simulink model "Control_test"  (R2014b)
settings: Solver=FixedStepDiscrete  StartTime=0.0  StopTime=Inf  FixedStep=0.001  RelTol=1e-3
PostLoadFcn:
  | , if any(exist('dsrtsu_mdlpostloadfcn', 'file') == [2, 3, 6]), try dsrtsu_mdlpostloadfcn('Execute', bdroot); catch fprintf('Error in PostLoadFcn (dsrtsu_mdlpostloadfcn) for model "%s":\n %s\n', bdroot, lasterr); end, end,
undefined symbols (not defined in the file or in its folder): dtLocal, slcm
libraries: rtican x163, simulink x14
(part 22 of 34)

== system Control_test/InputProcessing/RadarCanProcessing/Track24 ==
  Bus Creator : BusCreator  Inputs=12
  ESR_Track24 : rtican/RTICAN Receive (RX)   Reserved1=[]  Reserved2=[]  Reserved3=[]  Reserved4=[]  SfcnMessage=[]  Msg_Struct=[]  BoardTypeNo=[]  BoardNo=[]  ChannelNo=[]  Parameters=[]  DialogFcn=[]  UnitName=[]  Revision=[]  UnitValues=[]  DSProperties=struct('RTI',struct('Version',uint32(5),'BlockType',struct('isSLSource',uint8(1),'isSLSink',uint8(1),'isHWSource',uint8(0),'isHWSink',uint8(0),'isSetup',uint8(0),'isInline',uint8(1),'isNonInline',uint8(0),'isInterrupt',uint8(0),'isChannelwise',uint8(0)),'IOBoardType','RTICAN','UnitType','MESSAGE','Identifier','RX','DialogType','MSVC','BlockSet','RTICAN','SlaveProcessor','CAN'))  RTIBlockInterface=struct('OutputPortsWidth',int32([1 1 1 1 1 1 1 1 1 1 1 1]),'OutputPortsActive',[1 1 1 1 1 1 1 1 1 1 1 1],'OutputPortsName',{{'CAN_TX_TRACK_RANGE_RATE_24','CAN_TX_TRACK_MED_RANGE_MODE_24','CAN_TX_TRACK_RANGE_ACCEL_24','CAN_TX_TRACK_WIDTH_24','CAN_TX_TRACK_ROLLING_COUNT_24','CAN_TX_TRACK_BRIDGE_OBJECT_24','CAN_TX_TRACK_RANGE_24','CAN_TX_TRACK_ANGLE_24','CAN_TX_TRACK_STATUS_24','CAN_TX_TRACK_ONCOMING_24','CAN_TX_TRACK_GROUPING_CHANGED_24','CAN_TX_TRACK_LAT_RATE_24'}},'OutputPortsDataType',{{'SS_DOUBLE','SS_DOUBLE','SS_DOUBLE','SS_DOUBLE','SS_DOUBLE','SS_DOUBLE','SS_DOUBLE','SS_DOUBLE','SS_DOUBLE','SS_DOUBLE','SS_DOUBLE','SS_DOUBLE'}},'OutputPortsLabel',{{'CAN_TX_TRACK_RANGE_RATE_24','CAN_TX_TRACK_MED_RANGE_MODE_24','CAN_TX_TRACK_RANGE_ACCEL_24','CAN_TX_TRACK_WIDTH_24','CAN_TX_TRACK_ROLLING_COUNT_24','CAN_TX_TRACK_BRIDGE_OBJECT_24','CAN_TX_TRACK_RANGE_24','CAN_TX_TRACK_ANGLE_24','CAN_TX_TRACK_STATUS_24','CAN_TX_TRACK_ONCOMING_24','CAN_TX_TRACK_GROUPING_CHANGED_24','CAN_TX_TRACK_LAT_RATE_24'}},'OutputPortsLabelMode','ON','InputPortsWidth',int32(0),'InputPortsActive',0,'DialogFcn','rtican_message_interface_gui','BlockDisplay',{{'','center'}},'IconTransparency','on','ParameterTunableNames',{{}},'InitLevel',3,'BlockName',struct('Token',{{'ESR_Track24'}}),'SampleTime',{{0.01}},'TriggerPort',{{'none'}},'EnablePort',{{'none'}})  RTIBlockParameters=struct('BoardTypeNo',{{1,'OFF',[]}},'BoardNo',{{2,'ON',[1 16]}},'ChannelNo',{{2,'ON',[1 2]}},'Parameters',{{struct('DataFileSupport',struct('DataFileSelectedMaster',1,'DataFileSelectedLocal',0,'DataFileName','c:\users\mpc_car\documents\github\mpc-car\controller\dbcfiles\esr_dv3_64tgt.dbc|','DataFileDate',{{{['02-Nov-2012 20:32:52']},{['21-Mar-2013 13:39:53']},{['28-Sep-2011 17:08:52']}}},'SelectedFile',['<no file selected>'],'InterfaceFcn','rtican_dbc_file_parser'),'Options',struct('StatusSelected',0,'TimeSelected',0,'DeltaTimeSelected',0,'BytePortSelected',0,'MessageLengthSelected',0,'TriggerPort',struct('Selected',0,'TriggerType',0),'UserCoding',struct('Selected',0,'InterfaceFile','UserDecodingFile','FcnName','UserDecodeFcn','InportSelected',0,'InportWidth',1,'OutportSelected',0,'OutportWidth',1),'EnablePortSelected',0,'SignalOnPortnameSelected',1,'UseRXService',0),'Message',struct('MsgOnBlocknameSelected',1,'MsgName','ESR_Track24','MsgIdFormat',0,'MsgId',1303,'MsgLength',8,'NumSignals',12,'SampleTime',0.01,'Signal',struct('SgnName',{'CAN_TX_TRACK_RANGE_RATE_24','CAN_TX_TRACK_MED_RANGE_MODE_24','CAN_TX_TRACK_RANGE_ACCEL_24','CAN_TX_TRACK_WIDTH_24','CAN_TX_TRACK_ROLLING_COUNT_24','CAN_TX_TRACK_BRIDGE_OBJECT_24','CAN_TX_TRACK_RANGE_24','CAN_TX_TRACK_ANGLE_24','CAN_TX_TRACK_STATUS_24','CAN_TX_TRACK_ONCOMING_24','CAN_TX_TRACK_GROUPING_CHANGED_24','CAN_TX_TRACK_LAT_RATE_24'},'SgnStartBit',{0,14,16,26,30,31,32,43,53,56,57,58},'SgnLength',{14,2,10,4,1,1,11,10,3,1,1,6},'SgnType',{0,0,0,0,0,0,0,0,0,0,0,0},'ModeValue',{-1,-1,-1,-1,-1,-1,-1,-1,-1,-1,-1,-1},'DataType',{1,0,1,0,0,0,0,1,0,0,0,1},'ByteLayout',{2,2,2,2,2,2,2,2,2,2,2,2},'Factor',{0.01,1,0.05,0.5,1,1,0.1,0.1,1,1,1,0.25},'Offset',{0,0,0,0,0,0,0,0,0,0,0,0},'SgnComment',{{''},{''},{''},{''},{''},{''},{''},{''},{''},{''},{''},{''}},'SgnUnit',{'m/s','','m/s/s','m','','','m','deg','','','',''},'Min',{-81.92,0,-25.6,0,0,0,0,-51.2,0,0,0,-8},'Max',{81.91,3,25.55,7.5,1,0,204.7,51.1,7,0,0,7.75},'SLDataType',{'SS_DOUBLE','SS_DOUBLE','SS_DOUBLE','SS_DOUBLE','SS_DOUBLE','SS_DOUBLE','SS_DOUBLE','SS_DOUBLE','SS_DOUBLE','SS_DOUBLE','SS_DOUBLE','SS_DOUBLE'}),'MsgIdNumFormat',0,'MsgComment',{{''}}),'Version',1.2,'general',struct('isFromLib',0)),'OFF',[]}},'GroupId',{{struct('Group',{{'RTICAN'}},'No',4,'Behavior',{{'NAMECHANGE'}},'BlockType',{{'SINK'}},'NameChangeFlag',0),'OFF',[]}},'SFcnRTICANMessage',{{struct('MsgType','RX','SFcnPortType','Scalar','MsgName','ESR_Track24','MsgIdFormat','STD','MsgId',1303,'MsgLength',8,'NumSignals',12,'SampleTime',0.01,'Signal',struct('SgnName',{'CAN_TX_TRACK_RANGE_RATE_24','CAN_TX_TRACK_MED_RANGE_MODE_24','CAN_TX_TRACK_RANGE_ACCEL_24','CAN_TX_TRACK_WIDTH_24','CAN_TX_TRACK_ROLLING_COUNT_24','CAN_TX_TRACK_BRIDGE_OBJECT_24','CAN_TX_TRACK_RANGE_24','CAN_TX_TRACK_ANGLE_24','CAN_TX_TRACK_STATUS_24','CAN_TX_TRACK_ONCOMING_24','CAN_TX_TRACK_GROUPING_CHANGED_24','CAN_TX_TRACK_LAT_RATE_24'},'SgnStartBit',{0,14,16,26,30,31,32,43,53,56,57,58},'SgnLength',{14,2,10,4,1,1,11,10,3,1,1,6},'SgnType',{'standard','standard','standard','standard','standard','standard','standard','standard','standard','standard','standard','standard'},'ModeValue',{-1,-1,-1,-1,-1,-1,-1,-1,-1,-1,-1,-1},'DataType',{['signed int'],['unsigned int'],['signed int'],['unsigned int'],['unsigned int'],['unsigned int'],['unsigned int'],['signed int'],['unsigned int'],['unsigned int'],['unsigned int'],['signed int']},'ByteLayout',{['motorola back.'],['motorola back.'],['motorola back.'],['motorola back.'],['motorola back.'],['motorola back.'],['motorola back.'],['motorola back.'],['motorola back.'],['motorola back.'],['motorola back.'],['motorola back.']},'Factor',{0.01,1,0.05,0.5,1,1,0.1,0.1,1,1,1,0.25},'Offset',{0,0,0,0,0,0,0,0,0,0,0,0},'SLDataType',{'SS_DOUBLE','SS_DOUBLE','SS_DOUBLE','SS_DOUBLE','SS_DOUBLE','SS_DOUBLE','SS_DOUBLE','SS_DOUBLE','SS_DOUBLE','SS_DOUBLE','SS_DOUBLE','SS_DOUBLE'}),'StatusSelected','no','TimeSelected','no','DeltaTimeSelected','no','BytePortSelected','no','MessageLengthSelected','no','TriggerPort',struct('Selected','no','TriggerType',0),'UserCoding',struct('Selected','no','InterfaceFile','UserDecodingFile','FcnName','UserDecodeFcn','InportSelected','no','InportWidth',1,'OutportSelected','no','OutportWidth',1),'EnablePortSelected','no','UseRXService','no','BoardType','DS1','BoardNo',2,'ControllerNo',2),'OFF',[]}},'TLCFileName',{{'rtican_rx_message','OFF',[]}})  RTISFcnParameters=struct('SFcnRTICANMessage','struct','TLCFileName','char')  RTIBlockParaDefault=struct('BoardTypeNo',4302,'BoardNo',1,'ChannelNo',1,'Parameters',struct('DataFileSupport',struct('DataFileSelectedMaster',0,'DataFileSelectedLocal',0,'DataFileName','','DataFileDate','','SelectedFile',['<no file selected>']),'Options',struct('StatusSelected',1,'TimeSelected',1,'DeltaTimeSelected',1,'BytePortSelected',0,'MessageLengthSelected',0,'TriggerPort',struct('Selected',0,'TriggerType','rising'),'UserCoding',struct('Selected',0,'InterfaceFile','UserDecodingFile','FcnName','UserDecodeFcn','InportSelected',0,'InportWidth',1,'OutportSelected',0,'OutportWidth',1),'EnablePortSelected',0,'SignalOnPortnameSelected',1,'UseRXService',0),'Message',struct('MsgOnBlocknameSelected',0,'MsgName',['RX Message'],'MsgIdFormat',0,'MsgId',100,'MsgLength',8,'NumSignals',1,'SampleTime',-1,'Signal',struct('SgnName',['RX signal'],'SgnStartBit',0,'SgnLength',8,'SgnType',0,'ModeValue',-1,'DataType',0,'SLDataType','SS_DOUBLE','ByteLayout',0,'Factor',1,'Offset',0,'Min',0,'Max',255,'SgnComment',{{}},'SgnUnit',''),'MsgIdNumFormat',0,'MsgComment',{{''}}),'Version',1.2,'general',struct('isFromLib',1)),'GroupId',struct('Group',{{'RTICAN'}},'No',1,'Behavior',{{'NAMECHANGE'}},'BlockType',{{'SINK'}},'NameChangeFlag',0),'SFcnRTICANMessage',struct('MsgType','RX','MsgName',['RX Message'],'MsgIdFormat','STD','MsgId',100,'MsgLength',8,'NumSignals',1,'SampleTime',-1,'Signal',struct('SgnName',['RX signal'],'SgnStartBit',0,'SgnLength',8,'SgnType','standard','ModeValue',-1,'DataType',['unsigned int'],'ByteLayout',['little endian'],'SLDataType','SS_DOUBLE','Factor',1,'Offset',0),'StatusSelected','yes','TimeSelected','yes','DeltaTimeSelected','yes','BytePortSelected','no','MessageLengthSelected','no','EnablePortSelected','no','UserCoding',struct('Selected','no','InterfaceFile','UserDecodingFile','FcnName','UserDecodeFcn','InportSelected','no','InportWidth',1,'OutportSelected','no','OutportWidth',1),'TriggerPort',struct('Selected','no','TriggerType','rising'),'UseRXService','no','BoardType','DS4302','BoardNo',1,'ControllerNo',1,'SFcnPortType','Scalar'),'TLCFileName','rtican_rx_message')
      settings: AttributesFormatString=Group Id: RTICAN4\n
  Out1 : Outport
  wires:
  Bus Creator/1 -> Out1/1  "Track24"
  ESR_Track24/1 -> Bus Creator/1  "CAN_TX_TRACK_RANGE_RATE_24"
  ESR_Track24/2 -> Bus Creator/2  "CAN_TX_TRACK_MED_RANGE_MODE_24"
  ESR_Track24/3 -> Bus Creator/3  "CAN_TX_TRACK_RANGE_ACCEL_24"
  ESR_Track24/4 -> Bus Creator/4  "CAN_TX_TRACK_WIDTH_24"
  ESR_Track24/5 -> Bus Creator/5  "CAN_TX_TRACK_ROLLING_COUNT_24"
  ESR_Track24/6 -> Bus Creator/6  "CAN_TX_TRACK_BRIDGE_OBJECT_24"
  ESR_Track24/7 -> Bus Creator/7  "CAN_TX_TRACK_RANGE_24"
  ESR_Track24/8 -> Bus Creator/8  "CAN_TX_TRACK_ANGLE_24"
  ESR_Track24/9 -> Bus Creator/9  "CAN_TX_TRACK_STATUS_24"
  ESR_Track24/10 -> Bus Creator/10  "CAN_TX_TRACK_ONCOMING_24"
  ESR_Track24/11 -> Bus Creator/11  "CAN_TX_TRACK_GROUPING_CHANGED_24"
  ESR_Track24/12 -> Bus Creator/12  "CAN_TX_TRACK_LAT_RATE_24"

== system Control_test/InputProcessing/RadarCanProcessing/Track25 ==
  Bus Creator : BusCreator  Inputs=12
  ESR_Track25 : rtican/RTICAN Receive (RX)   Reserved1=[]  Reserved2=[]  Reserved3=[]  Reserved4=[]  SfcnMessage=[]  Msg_Struct=[]  BoardTypeNo=[]  BoardNo=[]  ChannelNo=[]  Parameters=[]  DialogFcn=[]  UnitName=[]  Revision=[]  UnitValues=[]  DSProperties=struct('RTI',struct('Version',uint32(5),'BlockType',struct('isSLSource',uint8(1),'isSLSink',uint8(1),'isHWSource',uint8(0),'isHWSink',uint8(0),'isSetup',uint8(0),'isInline',uint8(1),'isNonInline',uint8(0),'isInterrupt',uint8(0),'isChannelwise',uint8(0)),'IOBoardType','RTICAN','UnitType','MESSAGE','Identifier','RX','DialogType','MSVC','BlockSet','RTICAN','SlaveProcessor','CAN'))  RTIBlockInterface=struct('OutputPortsWidth',int32([1 1 1 1 1 1 1 1 1 1 1 1]),'OutputPortsActive',[1 1 1 1 1 1 1 1 1 1 1 1],'OutputPortsName',{{'CAN_TX_TRACK_RANGE_RATE_25','CAN_TX_TRACK_MED_RANGE_MODE_25','CAN_TX_TRACK_RANGE_ACCEL_25','CAN_TX_TRACK_WIDTH_25','CAN_TX_TRACK_ROLLING_COUNT_25','CAN_TX_TRACK_BRIDGE_OBJECT_25','CAN_TX_TRACK_RANGE_25','CAN_TX_TRACK_ANGLE_25','CAN_TX_TRACK_STATUS_25','CAN_TX_TRACK_ONCOMING_25','CAN_TX_TRACK_GROUPING_CHANGED_25','CAN_TX_TRACK_LAT_RATE_25'}},'OutputPortsDataType',{{'SS_DOUBLE','SS_DOUBLE','SS_DOUBLE','SS_DOUBLE','SS_DOUBLE','SS_DOUBLE','SS_DOUBLE','SS_DOUBLE','SS_DOUBLE','SS_DOUBLE','SS_DOUBLE','SS_DOUBLE'}},'OutputPortsLabel',{{'CAN_TX_TRACK_RANGE_RATE_25','CAN_TX_TRACK_MED_RANGE_MODE_25','CAN_TX_TRACK_RANGE_ACCEL_25','CAN_TX_TRACK_WIDTH_25','CAN_TX_TRACK_ROLLING_COUNT_25','CAN_TX_TRACK_BRIDGE_OBJECT_25','CAN_TX_TRACK_RANGE_25','CAN_TX_TRACK_ANGLE_25','CAN_TX_TRACK_STATUS_25','CAN_TX_TRACK_ONCOMING_25','CAN_TX_TRACK_GROUPING_CHANGED_25','CAN_TX_TRACK_LAT_RATE_25'}},'OutputPortsLabelMode','ON','InputPortsWidth',int32(0),'InputPortsActive',0,'DialogFcn','rtican_message_interface_gui','BlockDisplay',{{'','center'}},'IconTransparency','on','ParameterTunableNames',{{}},'InitLevel',3,'BlockName',struct('Token',{{'ESR_Track25'}}),'SampleTime',{{0.01}},'TriggerPort',{{'none'}},'EnablePort',{{'none'}})  RTIBlockParameters=struct('BoardTypeNo',{{1,'OFF',[]}},'BoardNo',{{2,'ON',[1 16]}},'ChannelNo',{{2,'ON',[1 2]}},'Parameters',{{struct('DataFileSupport',struct('DataFileSelectedMaster',1,'DataFileSelectedLocal',1,'DataFileName','c:\users\mpc_car\documents\github\mpc-car\controller\dbcfiles\esr_dv3_64tgt.dbc|','DataFileDate',['26-Aug-2014 13:16:21'],'SelectedFile','..\..\dbcfiles\esr_dv3_64tgt.dbc','InterfaceFcn','rtican_dbc_file_parser'),'Options',struct('StatusSelected',0,'TimeSelected',0,'DeltaTimeSelected',0,'BytePortSelected',0,'MessageLengthSelected',0,'TriggerPort',struct('Selected',0,'TriggerType',0),'UserCoding',struct('Selected',0,'InterfaceFile','UserDecodingFile','FcnName','UserDecodeFcn','InportSelected',0,'InportWidth',1,'OutportSelected',0,'OutportWidth',1),'EnablePortSelected',0,'SignalOnPortnameSelected',1,'UseRXService',0),'Message',struct('MsgOnBlocknameSelected',1,'MsgName','ESR_Track25','MsgIdFormat',0,'MsgId',1304,'MsgLength',8,'NumSignals',12,'SampleTime',0.01,'Signal',struct('SgnName',{'CAN_TX_TRACK_RANGE_RATE_25','CAN_TX_TRACK_MED_RANGE_MODE_25','CAN_TX_TRACK_RANGE_ACCEL_25','CAN_TX_TRACK_WIDTH_25','CAN_TX_TRACK_ROLLING_COUNT_25','CAN_TX_TRACK_BRIDGE_OBJECT_25','CAN_TX_TRACK_RANGE_25','CAN_TX_TRACK_ANGLE_25','CAN_TX_TRACK_STATUS_25','CAN_TX_TRACK_ONCOMING_25','CAN_TX_TRACK_GROUPING_CHANGED_25','CAN_TX_TRACK_LAT_RATE_25'},'SgnStartBit',{0,14,16,26,30,31,32,43,53,56,57,58},'SgnLength',{14,2,10,4,1,1,11,10,3,1,1,6},'ByteLayout',{2,2,2,2,2,2,2,2,2,2,2,2},'Factor',{0.01,1,0.05,0.5,1,1,0.1,0.1,1,1,1,0.25},'Offset',{0,0,0,0,0,0,0,0,0,0,0,0},'SgnComment',{'','','','','','','','','','','',''},'SgnUnit',{'m/s','','m/s/s','m','','','m','deg','','','',''},'Min',{-81.92,0,-25.6,0,0,0,0,-51.2,0,0,0,-8},'Max',{81.91,3,25.55,7.5,1,0,204.7,51.1,7,0,0,7.75},'SgnType',{0,0,0,0,0,0,0,0,0,0,0,0},'SLDataType',{'SS_DOUBLE','SS_DOUBLE','SS_DOUBLE','SS_DOUBLE','SS_DOUBLE','SS_DOUBLE','SS_DOUBLE','SS_DOUBLE','SS_DOUBLE','SS_DOUBLE','SS_DOUBLE','SS_DOUBLE'},'DataType',{1,0,1,0,0,0,0,1,0,0,0,1},'ModeValue',{-1,-1,-1,-1,-1,-1,-1,-1,-1,-1,-1,-1}),'MsgIdNumFormat',0,'MsgComment',{{''}}),'Version',1.2,'general',struct('isFromLib',0)),'OFF',[]}},'GroupId',{{struct('Group',{{'RTICAN'}},'No',4,'Behavior',{{'NAMECHANGE'}},'BlockType',{{'SINK'}},'NameChangeFlag',0),'OFF',[]}},'SFcnRTICANMessage',{{struct('MsgType','RX','SFcnPortType','Scalar','MsgName','ESR_Track25','MsgIdFormat','STD','MsgId',1304,'MsgLength',8,'NumSignals',12,'SampleTime',0.01,'Signal',struct('SgnName',{'CAN_TX_TRACK_RANGE_RATE_25','CAN_TX_TRACK_MED_RANGE_MODE_25','CAN_TX_TRACK_RANGE_ACCEL_25','CAN_TX_TRACK_WIDTH_25','CAN_TX_TRACK_ROLLING_COUNT_25','CAN_TX_TRACK_BRIDGE_OBJECT_25','CAN_TX_TRACK_RANGE_25','CAN_TX_TRACK_ANGLE_25','CAN_TX_TRACK_STATUS_25','CAN_TX_TRACK_ONCOMING_25','CAN_TX_TRACK_GROUPING_CHANGED_25','CAN_TX_TRACK_LAT_RATE_25'},'SgnStartBit',{0,14,16,26,30,31,32,43,53,56,57,58},'SgnLength',{14,2,10,4,1,1,11,10,3,1,1,6},'ByteLayout',{['motorola back.'],['motorola back.'],['motorola back.'],['motorola back.'],['motorola back.'],['motorola back.'],['motorola back.'],['motorola back.'],['motorola back.'],['motorola back.'],['motorola back.'],['motorola back.']},'Factor',{0.01,1,0.05,0.5,1,1,0.1,0.1,1,1,1,0.25},'Offset',{0,0,0,0,0,0,0,0,0,0,0,0},'SgnType',{'standard','standard','standard','standard','standard','standard','standard','standard','standard','standard','standard','standard'},'SLDataType',{'SS_DOUBLE','SS_DOUBLE','SS_DOUBLE','SS_DOUBLE','SS_DOUBLE','SS_DOUBLE','SS_DOUBLE','SS_DOUBLE','SS_DOUBLE','SS_DOUBLE','SS_DOUBLE','SS_DOUBLE'},'DataType',{['signed int'],['unsigned int'],['signed int'],['unsigned int'],['unsigned int'],['unsigned int'],['unsigned int'],['signed int'],['unsigned int'],['unsigned int'],['unsigned int'],['signed int']},'ModeValue',{-1,-1,-1,-1,-1,-1,-1,-1,-1,-1,-1,-1}),'StatusSelected','no','TimeSelected','no','DeltaTimeSelected','no','BytePortSelected','no','MessageLengthSelected','no','TriggerPort',struct('Selected','no','TriggerType',0),'UserCoding',struct('Selected','no','InterfaceFile','UserDecodingFile','FcnName','UserDecodeFcn','InportSelected','no','InportWidth',1,'OutportSelected','no','OutportWidth',1),'EnablePortSelected','no','UseRXService','no','BoardType','DS1','BoardNo',2,'ControllerNo',2),'OFF',[]}},'TLCFileName',{{'rtican_rx_message','OFF',[]}})  RTISFcnParameters=struct('SFcnRTICANMessage','struct','TLCFileName','char')  RTIBlockParaDefault=struct('BoardTypeNo',4302,'BoardNo',1,'ChannelNo',1,'Parameters',struct('DataFileSupport',struct('DataFileSelectedMaster',0,'DataFileSelectedLocal',0,'DataFileName','','DataFileDate','','SelectedFile',['<no file selected>']),'Options',struct('StatusSelected',1,'TimeSelected',1,'DeltaTimeSelected',1,'BytePortSelected',0,'MessageLengthSelected',0,'TriggerPort',struct('Selected',0,'TriggerType','rising'),'UserCoding',struct('Selected',0,'InterfaceFile','UserDecodingFile','FcnName','UserDecodeFcn','InportSelected',0,'InportWidth',1,'OutportSelected',0,'OutportWidth',1),'EnablePortSelected',0,'SignalOnPortnameSelected',1,'UseRXService',0),'Message',struct('MsgOnBlocknameSelected',0,'MsgName',['RX Message'],'MsgIdFormat',0,'MsgId',100,'MsgLength',8,'NumSignals',1,'SampleTime',-1,'Signal',struct('SgnName',['RX signal'],'SgnStartBit',0,'SgnLength',8,'SgnType',0,'ModeValue',-1,'DataType',0,'SLDataType','SS_DOUBLE','ByteLayout',0,'Factor',1,'Offset',0,'Min',0,'Max',255,'SgnComment',{{}},'SgnUnit',''),'MsgIdNumFormat',0,'MsgComment',{{''}}),'Version',1.2,'general',struct('isFromLib',1)),'GroupId',struct('Group',{{'RTICAN'}},'No',1,'Behavior',{{'NAMECHANGE'}},'BlockType',{{'SINK'}},'NameChangeFlag',0),'SFcnRTICANMessage',struct('MsgType','RX','MsgName',['RX Message'],'MsgIdFormat','STD','MsgId',100,'MsgLength',8,'NumSignals',1,'SampleTime',-1,'Signal',struct('SgnName',['RX signal'],'SgnStartBit',0,'SgnLength',8,'SgnType','standard','ModeValue',-1,'DataType',['unsigned int'],'ByteLayout',['little endian'],'SLDataType','SS_DOUBLE','Factor',1,'Offset',0),'StatusSelected','yes','TimeSelected','yes','DeltaTimeSelected','yes','BytePortSelected','no','MessageLengthSelected','no','EnablePortSelected','no','UserCoding',struct('Selected','no','InterfaceFile','UserDecodingFile','FcnName','UserDecodeFcn','InportSelected','no','InportWidth',1,'OutportSelected','no','OutportWidth',1),'TriggerPort',struct('Selected','no','TriggerType','rising'),'UseRXService','no','BoardType','DS4302','BoardNo',1,'ControllerNo',1,'SFcnPortType','Scalar'),'TLCFileName','rtican_rx_message')
      settings: AttributesFormatString=Group Id: RTICAN4\n
  Out1 : Outport
  wires:
  Bus Creator/1 -> Out1/1  "Track25"
  ESR_Track25/1 -> Bus Creator/1  "CAN_TX_TRACK_RANGE_RATE_25"
  ESR_Track25/2 -> Bus Creator/2  "CAN_TX_TRACK_MED_RANGE_MODE_25"
  ESR_Track25/3 -> Bus Creator/3  "CAN_TX_TRACK_RANGE_ACCEL_25"
  ESR_Track25/4 -> Bus Creator/4  "CAN_TX_TRACK_WIDTH_25"
  ESR_Track25/5 -> Bus Creator/5  "CAN_TX_TRACK_ROLLING_COUNT_25"
  ESR_Track25/6 -> Bus Creator/6  "CAN_TX_TRACK_BRIDGE_OBJECT_25"
  ESR_Track25/7 -> Bus Creator/7  "CAN_TX_TRACK_RANGE_25"
  ESR_Track25/8 -> Bus Creator/8  "CAN_TX_TRACK_ANGLE_25"
  ESR_Track25/9 -> Bus Creator/9  "CAN_TX_TRACK_STATUS_25"
  ESR_Track25/10 -> Bus Creator/10  "CAN_TX_TRACK_ONCOMING_25"
  ESR_Track25/11 -> Bus Creator/11  "CAN_TX_TRACK_GROUPING_CHANGED_25"
  ESR_Track25/12 -> Bus Creator/12  "CAN_TX_TRACK_LAT_RATE_25"

== system Control_test/InputProcessing/RadarCanProcessing/Track26 ==
  Bus Creator : BusCreator  Inputs=12
  ESR_Track26 : rtican/RTICAN Receive (RX)   Reserved1=[]  Reserved2=[]  Reserved3=[]  Reserved4=[]  SfcnMessage=[]  Msg_Struct=[]  BoardTypeNo=[]  BoardNo=[]  ChannelNo=[]  Parameters=[]  DialogFcn=[]  UnitName=[]  Revision=[]  UnitValues=[]  DSProperties=struct('RTI',struct('Version',uint32(5),'BlockType',struct('isSLSource',uint8(1),'isSLSink',uint8(1),'isHWSource',uint8(0),'isHWSink',uint8(0),'isSetup',uint8(0),'isInline',uint8(1),'isNonInline',uint8(0),'isInterrupt',uint8(0),'isChannelwise',uint8(0)),'IOBoardType','RTICAN','UnitType','MESSAGE','Identifier','RX','DialogType','MSVC','BlockSet','RTICAN','SlaveProcessor','CAN'))  RTIBlockInterface=struct('OutputPortsWidth',int32([1 1 1 1 1 1 1 1 1 1 1 1]),'OutputPortsActive',[1 1 1 1 1 1 1 1 1 1 1 1],'OutputPortsName',{{'CAN_TX_TRACK_RANGE_RATE_26','CAN_TX_TRACK_MED_RANGE_MODE_26','CAN_TX_TRACK_RANGE_ACCEL_26','CAN_TX_TRACK_WIDTH_26','CAN_TX_TRACK_ROLLING_COUNT_26','CAN_TX_TRACK_BRIDGE_OBJECT_26','CAN_TX_TRACK_RANGE_26','CAN_TX_TRACK_ANGLE_26','CAN_TX_TRACK_STATUS_26','CAN_TX_TRACK_ONCOMING_26','CAN_TX_TRACK_GROUPING_CHANGED_26','CAN_TX_TRACK_LAT_RATE_26'}},'OutputPortsDataType',{{'SS_DOUBLE','SS_DOUBLE','SS_DOUBLE','SS_DOUBLE','SS_DOUBLE','SS_DOUBLE','SS_DOUBLE','SS_DOUBLE','SS_DOUBLE','SS_DOUBLE','SS_DOUBLE','SS_DOUBLE'}},'OutputPortsLabel',{{'CAN_TX_TRACK_RANGE_RATE_26','CAN_TX_TRACK_MED_RANGE_MODE_26','CAN_TX_TRACK_RANGE_ACCEL_26','CAN_TX_TRACK_WIDTH_26','CAN_TX_TRACK_ROLLING_COUNT_26','CAN_TX_TRACK_BRIDGE_OBJECT_26','CAN_TX_TRACK_RANGE_26','CAN_TX_TRACK_ANGLE_26','CAN_TX_TRACK_STATUS_26','CAN_TX_TRACK_ONCOMING_26','CAN_TX_TRACK_GROUPING_CHANGED_26','CAN_TX_TRACK_LAT_RATE_26'}},'OutputPortsLabelMode','ON','InputPortsWidth',int32(0),'InputPortsActive',0,'DialogFcn','rtican_message_interface_gui','BlockDisplay',{{'','center'}},'IconTransparency','on','ParameterTunableNames',{{}},'InitLevel',3,'BlockName',struct('Token',{{'ESR_Track26'}}),'SampleTime',{{0.01}},'TriggerPort',{{'none'}},'EnablePort',{{'none'}})  RTIBlockParameters=struct('BoardTypeNo',{{1,'OFF',[]}},'BoardNo',{{2,'ON',[1 16]}},'ChannelNo',{{2,'ON',[1 2]}},'Parameters',{{struct('DataFileSupport',struct('DataFileSelectedMaster',1,'DataFileSelectedLocal',0,'DataFileName','c:\users\mpc_car\documents\github\mpc-car\controller\dbcfiles\esr_dv3_64tgt.dbc|','DataFileDate',{{{['02-Nov-2012 20:32:52']},{['21-Mar-2013 13:39:53']},{['28-Sep-2011 17:08:52']}}},'SelectedFile',['<no file selected>'],'InterfaceFcn','rtican_dbc_file_parser'),'Options',struct('StatusSelected',0,'TimeSelected',0,'DeltaTimeSelected',0,'BytePortSelected',0,'MessageLengthSelected',0,'TriggerPort',struct('Selected',0,'TriggerType',0),'UserCoding',struct('Selected',0,'InterfaceFile','UserDecodingFile','FcnName','UserDecodeFcn','InportSelected',0,'InportWidth',1,'OutportSelected',0,'OutportWidth',1),'EnablePortSelected',0,'SignalOnPortnameSelected',1,'UseRXService',0),'Message',struct('MsgOnBlocknameSelected',1,'MsgName','ESR_Track26','MsgIdFormat',0,'MsgId',1305,'MsgLength',8,'NumSignals',12,'SampleTime',0.01,'Signal',struct('SgnName',{'CAN_TX_TRACK_RANGE_RATE_26','CAN_TX_TRACK_MED_RANGE_MODE_26','CAN_TX_TRACK_RANGE_ACCEL_26','CAN_TX_TRACK_WIDTH_26','CAN_TX_TRACK_ROLLING_COUNT_26','CAN_TX_TRACK_BRIDGE_OBJECT_26','CAN_TX_TRACK_RANGE_26','CAN_TX_TRACK_ANGLE_26','CAN_TX_TRACK_STATUS_26','CAN_TX_TRACK_ONCOMING_26','CAN_TX_TRACK_GROUPING_CHANGED_26','CAN_TX_TRACK_LAT_RATE_26'},'SgnStartBit',{0,14,16,26,30,31,32,43,53,56,57,58},'SgnLength',{14,2,10,4,1,1,11,10,3,1,1,6},'SgnType',{0,0,0,0,0,0,0,0,0,0,0,0},'ModeValue',{-1,-1,-1,-1,-1,-1,-1,-1,-1,-1,-1,-1},'DataType',{1,0,1,0,0,0,0,1,0,0,0,1},'ByteLayout',{2,2,2,2,2,2,2,2,2,2,2,2},'Factor',{0.01,1,0.05,0.5,1,1,0.1,0.1,1,1,1,0.25},'Offset',{0,0,0,0,0,0,0,0,0,0,0,0},'SgnComment',{{''},{''},{''},{''},{''},{''},{''},{''},{''},{''},{''},{''}},'SgnUnit',{'m/s','','m/s/s','m','','','m','deg','','','',''},'Min',{-81.92,0,-25.6,0,0,0,0,-51.2,0,0,0,-8},'Max',{81.91,3,25.55,7.5,1,0,204.7,51.1,7,0,0,7.75},'SLDataType',{'SS_DOUBLE','SS_DOUBLE','SS_DOUBLE','SS_DOUBLE','SS_DOUBLE','SS_DOUBLE','SS_DOUBLE','SS_DOUBLE','SS_DOUBLE','SS_DOUBLE','SS_DOUBLE','SS_DOUBLE'}),'MsgIdNumFormat',0,'MsgComment',{{''}}),'Version',1.2,'general',struct('isFromLib',0)),'OFF',[]}},'GroupId',{{struct('Group',{{'RTICAN'}},'No',4,'Behavior',{{'NAMECHANGE'}},'BlockType',{{'SINK'}},'NameChangeFlag',0),'OFF',[]}},'SFcnRTICANMessage',{{struct('MsgType','RX','SFcnPortType','Scalar','MsgName','ESR_Track26','MsgIdFormat','STD','MsgId',1305,'MsgLength',8,'NumSignals',12,'SampleTime',0.01,'Signal',struct('SgnName',{'CAN_TX_TRACK_RANGE_RATE_26','CAN_TX_TRACK_MED_RANGE_MODE_26','CAN_TX_TRACK_RANGE_ACCEL_26','CAN_TX_TRACK_WIDTH_26','CAN_TX_TRACK_ROLLING_COUNT_26','CAN_TX_TRACK_BRIDGE_OBJECT_26','CAN_TX_TRACK_RANGE_26','CAN_TX_TRACK_ANGLE_26','CAN_TX_TRACK_STATUS_26','CAN_TX_TRACK_ONCOMING_26','CAN_TX_TRACK_GROUPING_CHANGED_26','CAN_TX_TRACK_LAT_RATE_26'},'SgnStartBit',{0,14,16,26,30,31,32,43,53,56,57,58},'SgnLength',{14,2,10,4,1,1,11,10,3,1,1,6},'SgnType',{'standard','standard','standard','standard','standard','standard','standard','standard','standard','standard','standard','standard'},'ModeValue',{-1,-1,-1,-1,-1,-1,-1,-1,-1,-1,-1,-1},'DataType',{['signed int'],['unsigned int'],['signed int'],['unsigned int'],['unsigned int'],['unsigned int'],['unsigned int'],['signed int'],['unsigned int'],['unsigned int'],['unsigned int'],['signed int']},'ByteLayout',{['motorola back.'],['motorola back.'],['motorola back.'],['motorola back.'],['motorola back.'],['motorola back.'],['motorola back.'],['motorola back.'],['motorola back.'],['motorola back.'],['motorola back.'],['motorola back.']},'Factor',{0.01,1,0.05,0.5,1,1,0.1,0.1,1,1,1,0.25},'Offset',{0,0,0,0,0,0,0,0,0,0,0,0},'SLDataType',{'SS_DOUBLE','SS_DOUBLE','SS_DOUBLE','SS_DOUBLE','SS_DOUBLE','SS_DOUBLE','SS_DOUBLE','SS_DOUBLE','SS_DOUBLE','SS_DOUBLE','SS_DOUBLE','SS_DOUBLE'}),'StatusSelected','no','TimeSelected','no','DeltaTimeSelected','no','BytePortSelected','no','MessageLengthSelected','no','TriggerPort',struct('Selected','no','TriggerType',0),'UserCoding',struct('Selected','no','InterfaceFile','UserDecodingFile','FcnName','UserDecodeFcn','InportSelected','no','InportWidth',1,'OutportSelected','no','OutportWidth',1),'EnablePortSelected','no','UseRXService','no','BoardType','DS1','BoardNo',2,'ControllerNo',2),'OFF',[]}},'TLCFileName',{{'rtican_rx_message','OFF',[]}})  RTISFcnParameters=struct('SFcnRTICANMessage','struct','TLCFileName','char')  RTIBlockParaDefault=struct('BoardTypeNo',4302,'BoardNo',1,'ChannelNo',1,'Parameters',struct('DataFileSupport',struct('DataFileSelectedMaster',0,'DataFileSelectedLocal',0,'DataFileName','','DataFileDate','','SelectedFile',['<no file selected>']),'Options',struct('StatusSelected',1,'TimeSelected',1,'DeltaTimeSelected',1,'BytePortSelected',0,'MessageLengthSelected',0,'TriggerPort',struct('Selected',0,'TriggerType','rising'),'UserCoding',struct('Selected',0,'InterfaceFile','UserDecodingFile','FcnName','UserDecodeFcn','InportSelected',0,'InportWidth',1,'OutportSelected',0,'OutportWidth',1),'EnablePortSelected',0,'SignalOnPortnameSelected',1,'UseRXService',0),'Message',struct('MsgOnBlocknameSelected',0,'MsgName',['RX Message'],'MsgIdFormat',0,'MsgId',100,'MsgLength',8,'NumSignals',1,'SampleTime',-1,'Signal',struct('SgnName',['RX signal'],'SgnStartBit',0,'SgnLength',8,'SgnType',0,'ModeValue',-1,'DataType',0,'SLDataType','SS_DOUBLE','ByteLayout',0,'Factor',1,'Offset',0,'Min',0,'Max',255,'SgnComment',{{}},'SgnUnit',''),'MsgIdNumFormat',0,'MsgComment',{{''}}),'Version',1.2,'general',struct('isFromLib',1)),'GroupId',struct('Group',{{'RTICAN'}},'No',1,'Behavior',{{'NAMECHANGE'}},'BlockType',{{'SINK'}},'NameChangeFlag',0),'SFcnRTICANMessage',struct('MsgType','RX','MsgName',['RX Message'],'MsgIdFormat','STD','MsgId',100,'MsgLength',8,'NumSignals',1,'SampleTime',-1,'Signal',struct('SgnName',['RX signal'],'SgnStartBit',0,'SgnLength',8,'SgnType','standard','ModeValue',-1,'DataType',['unsigned int'],'ByteLayout',['little endian'],'SLDataType','SS_DOUBLE','Factor',1,'Offset',0),'StatusSelected','yes','TimeSelected','yes','DeltaTimeSelected','yes','BytePortSelected','no','MessageLengthSelected','no','EnablePortSelected','no','UserCoding',struct('Selected','no','InterfaceFile','UserDecodingFile','FcnName','UserDecodeFcn','InportSelected','no','InportWidth',1,'OutportSelected','no','OutportWidth',1),'TriggerPort',struct('Selected','no','TriggerType','rising'),'UseRXService','no','BoardType','DS4302','BoardNo',1,'ControllerNo',1,'SFcnPortType','Scalar'),'TLCFileName','rtican_rx_message')
      settings: AttributesFormatString=Group Id: RTICAN4\n
  Out1 : Outport
  wires:
  Bus Creator/1 -> Out1/1  "Track26"
  ESR_Track26/1 -> Bus Creator/1  "CAN_TX_TRACK_RANGE_RATE_26"
  ESR_Track26/2 -> Bus Creator/2  "CAN_TX_TRACK_MED_RANGE_MODE_26"
  ESR_Track26/3 -> Bus Creator/3  "CAN_TX_TRACK_RANGE_ACCEL_26"
  ESR_Track26/4 -> Bus Creator/4  "CAN_TX_TRACK_WIDTH_26"
  ESR_Track26/5 -> Bus Creator/5  "CAN_TX_TRACK_ROLLING_COUNT_26"
  ESR_Track26/6 -> Bus Creator/6  "CAN_TX_TRACK_BRIDGE_OBJECT_26"
  ESR_Track26/7 -> Bus Creator/7  "CAN_TX_TRACK_RANGE_26"
  ESR_Track26/8 -> Bus Creator/8  "CAN_TX_TRACK_ANGLE_26"
  ESR_Track26/9 -> Bus Creator/9  "CAN_TX_TRACK_STATUS_26"
  ESR_Track26/10 -> Bus Creator/10  "CAN_TX_TRACK_ONCOMING_26"
  ESR_Track26/11 -> Bus Creator/11  "CAN_TX_TRACK_GROUPING_CHANGED_26"
  ESR_Track26/12 -> Bus Creator/12  "CAN_TX_TRACK_LAT_RATE_26"

== system Control_test/InputProcessing/RadarCanProcessing/Track27 ==
  Bus Creator : BusCreator  Inputs=12
  ESR_Track27 : rtican/RTICAN Receive (RX)   Reserved1=[]  Reserved2=[]  Reserved3=[]  Reserved4=[]  SfcnMessage=[]  Msg_Struct=[]  BoardTypeNo=[]  BoardNo=[]  ChannelNo=[]  Parameters=[]  DialogFcn=[]  UnitName=[]  Revision=[]  UnitValues=[]  DSProperties=struct('RTI',struct('Version',uint32(5),'BlockType',struct('isSLSource',uint8(1),'isSLSink',uint8(1),'isHWSource',uint8(0),'isHWSink',uint8(0),'isSetup',uint8(0),'isInline',uint8(1),'isNonInline',uint8(0),'isInterrupt',uint8(0),'isChannelwise',uint8(0)),'IOBoardType','RTICAN','UnitType','MESSAGE','Identifier','RX','DialogType','MSVC','BlockSet','RTICAN','SlaveProcessor','CAN'))  RTIBlockInterface=struct('OutputPortsWidth',int32([1 1 1 1 1 1 1 1 1 1 1 1]),'OutputPortsActive',[1 1 1 1 1 1 1 1 1 1 1 1],'OutputPortsName',{{'CAN_TX_TRACK_RANGE_RATE_27','CAN_TX_TRACK_MED_RANGE_MODE_27','CAN_TX_TRACK_RANGE_ACCEL_27','CAN_TX_TRACK_WIDTH_27','CAN_TX_TRACK_ROLLING_COUNT_27','CAN_TX_TRACK_BRIDGE_OBJECT_27','CAN_TX_TRACK_RANGE_27','CAN_TX_TRACK_ANGLE_27','CAN_TX_TRACK_STATUS_27','CAN_TX_TRACK_ONCOMING_27','CAN_TX_TRACK_GROUPING_CHANGED_27','CAN_TX_TRACK_LAT_RATE_27'}},'OutputPortsDataType',{{'SS_DOUBLE','SS_DOUBLE','SS_DOUBLE','SS_DOUBLE','SS_DOUBLE','SS_DOUBLE','SS_DOUBLE','SS_DOUBLE','SS_DOUBLE','SS_DOUBLE','SS_DOUBLE','SS_DOUBLE'}},'OutputPortsLabel',{{'CAN_TX_TRACK_RANGE_RATE_27','CAN_TX_TRACK_MED_RANGE_MODE_27','CAN_TX_TRACK_RANGE_ACCEL_27','CAN_TX_TRACK_WIDTH_27','CAN_TX_TRACK_ROLLING_COUNT_27','CAN_TX_TRACK_BRIDGE_OBJECT_27','CAN_TX_TRACK_RANGE_27','CAN_TX_TRACK_ANGLE_27','CAN_TX_TRACK_STATUS_27','CAN_TX_TRACK_ONCOMING_27','CAN_TX_TRACK_GROUPING_CHANGED_27','CAN_TX_TRACK_LAT_RATE_27'}},'OutputPortsLabelMode','ON','InputPortsWidth',int32(0),'InputPortsActive',0,'DialogFcn','rtican_message_interface_gui','BlockDisplay',{{'','center'}},'IconTransparency','on','ParameterTunableNames',{{}},'InitLevel',3,'BlockName',struct('Token',{{'ESR_Track27'}}),'SampleTime',{{0.01}},'TriggerPort',{{'none'}},'EnablePort',{{'none'}})  RTIBlockParameters=struct('BoardTypeNo',{{1,'OFF',[]}},'BoardNo',{{2,'ON',[1 16]}},'ChannelNo',{{2,'ON',[1 2]}},'Parameters',{{struct('DataFileSupport',struct('DataFileSelectedMaster',1,'DataFileSelectedLocal',0,'DataFileName','c:\users\mpc_car\documents\github\mpc-car\controller\dbcfiles\esr_dv3_64tgt.dbc|','DataFileDate',{{{['02-Nov-2012 20:32:52']},{['21-Mar-2013 13:39:53']},{['28-Sep-2011 17:08:52']}}},'SelectedFile',['<no file selected>'],'InterfaceFcn','rtican_dbc_file_parser'),'Options',struct('StatusSelected',0,'TimeSelected',0,'DeltaTimeSelected',0,'BytePortSelected',0,'MessageLengthSelected',0,'TriggerPort',struct('Selected',0,'TriggerType',0),'UserCoding',struct('Selected',0,'InterfaceFile','UserDecodingFile','FcnName','UserDecodeFcn','InportSelected',0,'InportWidth',1,'OutportSelected',0,'OutportWidth',1),'EnablePortSelected',0,'SignalOnPortnameSelected',1,'UseRXService',0),'Message',struct('MsgOnBlocknameSelected',1,'MsgName','ESR_Track27','MsgIdFormat',0,'MsgId',1306,'MsgLength',8,'NumSignals',12,'SampleTime',0.01,'Signal',struct('SgnName',{'CAN_TX_TRACK_RANGE_RATE_27','CAN_TX_TRACK_MED_RANGE_MODE_27','CAN_TX_TRACK_RANGE_ACCEL_27','CAN_TX_TRACK_WIDTH_27','CAN_TX_TRACK_ROLLING_COUNT_27','CAN_TX_TRACK_BRIDGE_OBJECT_27','CAN_TX_TRACK_RANGE_27','CAN_TX_TRACK_ANGLE_27','CAN_TX_TRACK_STATUS_27','CAN_TX_TRACK_ONCOMING_27','CAN_TX_TRACK_GROUPING_CHANGED_27','CAN_TX_TRACK_LAT_RATE_27'},'SgnStartBit',{0,14,16,26,30,31,32,43,53,56,57,58},'SgnLength',{14,2,10,4,1,1,11,10,3,1,1,6},'SgnType',{0,0,0,0,0,0,0,0,0,0,0,0},'ModeValue',{-1,-1,-1,-1,-1,-1,-1,-1,-1,-1,-1,-1},'DataType',{1,0,1,0,0,0,0,1,0,0,0,1},'ByteLayout',{2,2,2,2,2,2,2,2,2,2,2,2},'Factor',{0.01,1,0.05,0.5,1,1,0.1,0.1,1,1,1,0.25},'Offset',{0,0,0,0,0,0,0,0,0,0,0,0},'SgnComment',{{''},{''},{''},{''},{''},{''},{''},{''},{''},{''},{''},{''}},'SgnUnit',{'m/s','','m/s/s','m','','','m','deg','','','',''},'Min',{-81.92,0,-25.6,0,0,0,0,-51.2,0,0,0,-8},'Max',{81.91,3,25.55,7.5,1,0,204.7,51.1,7,0,0,7.75},'SLDataType',{'SS_DOUBLE','SS_DOUBLE','SS_DOUBLE','SS_DOUBLE','SS_DOUBLE','SS_DOUBLE','SS_DOUBLE','SS_DOUBLE','SS_DOUBLE','SS_DOUBLE','SS_DOUBLE','SS_DOUBLE'}),'MsgIdNumFormat',0,'MsgComment',{{''}}),'Version',1.2,'general',struct('isFromLib',0)),'OFF',[]}},'GroupId',{{struct('Group',{{'RTICAN'}},'No',4,'Behavior',{{'NAMECHANGE'}},'BlockType',{{'SINK'}},'NameChangeFlag',0),'OFF',[]}},'SFcnRTICANMessage',{{struct('MsgType','RX','SFcnPortType','Scalar','MsgName','ESR_Track27','MsgIdFormat','STD','MsgId',1306,'MsgLength',8,'NumSignals',12,'SampleTime',0.01,'Signal',struct('SgnName',{'CAN_TX_TRACK_RANGE_RATE_27','CAN_TX_TRACK_MED_RANGE_MODE_27','CAN_TX_TRACK_RANGE_ACCEL_27','CAN_TX_TRACK_WIDTH_27','CAN_TX_TRACK_ROLLING_COUNT_27','CAN_TX_TRACK_BRIDGE_OBJECT_27','CAN_TX_TRACK_RANGE_27','CAN_TX_TRACK_ANGLE_27','CAN_TX_TRACK_STATUS_27','CAN_TX_TRACK_ONCOMING_27','CAN_TX_TRACK_GROUPING_CHANGED_27','CAN_TX_TRACK_LAT_RATE_27'},'SgnStartBit',{0,14,16,26,30,31,32,43,53,56,57,58},'SgnLength',{14,2,10,4,1,1,11,10,3,1,1,6},'SgnType',{'standard','standard','standard','standard','standard','standard','standard','standard','standard','standard','standard','standard'},'ModeValue',{-1,-1,-1,-1,-1,-1,-1,-1,-1,-1,-1,-1},'DataType',{['signed int'],['unsigned int'],['signed int'],['unsigned int'],['unsigned int'],['unsigned int'],['unsigned int'],['signed int'],['unsigned int'],['unsigned int'],['unsigned int'],['signed int']},'ByteLayout',{['motorola back.'],['motorola back.'],['motorola back.'],['motorola back.'],['motorola back.'],['motorola back.'],['motorola back.'],['motorola back.'],['motorola back.'],['motorola back.'],['motorola back.'],['motorola back.']},'Factor',{0.01,1,0.05,0.5,1,1,0.1,0.1,1,1,1,0.25},'Offset',{0,0,0,0,0,0,0,0,0,0,0,0},'SLDataType',{'SS_DOUBLE','SS_DOUBLE','SS_DOUBLE','SS_DOUBLE','SS_DOUBLE','SS_DOUBLE','SS_DOUBLE','SS_DOUBLE','SS_DOUBLE','SS_DOUBLE','SS_DOUBLE','SS_DOUBLE'}),'StatusSelected','no','TimeSelected','no','DeltaTimeSelected','no','BytePortSelected','no','MessageLengthSelected','no','TriggerPort',struct('Selected','no','TriggerType',0),'UserCoding',struct('Selected','no','InterfaceFile','UserDecodingFile','FcnName','UserDecodeFcn','InportSelected','no','InportWidth',1,'OutportSelected','no','OutportWidth',1),'EnablePortSelected','no','UseRXService','no','BoardType','DS1','BoardNo',2,'ControllerNo',2),'OFF',[]}},'TLCFileName',{{'rtican_rx_message','OFF',[]}})  RTISFcnParameters=struct('SFcnRTICANMessage','struct','TLCFileName','char')  RTIBlockParaDefault=struct('BoardTypeNo',4302,'BoardNo',1,'ChannelNo',1,'Parameters',struct('DataFileSupport',struct('DataFileSelectedMaster',0,'DataFileSelectedLocal',0,'DataFileName','','DataFileDate','','SelectedFile',['<no file selected>']),'Options',struct('StatusSelected',1,'TimeSelected',1,'DeltaTimeSelected',1,'BytePortSelected',0,'MessageLengthSelected',0,'TriggerPort',struct('Selected',0,'TriggerType','rising'),'UserCoding',struct('Selected',0,'InterfaceFile','UserDecodingFile','FcnName','UserDecodeFcn','InportSelected',0,'InportWidth',1,'OutportSelected',0,'OutportWidth',1),'EnablePortSelected',0,'SignalOnPortnameSelected',1,'UseRXService',0),'Message',struct('MsgOnBlocknameSelected',0,'MsgName',['RX Message'],'MsgIdFormat',0,'MsgId',100,'MsgLength',8,'NumSignals',1,'SampleTime',-1,'Signal',struct('SgnName',['RX signal'],'SgnStartBit',0,'SgnLength',8,'SgnType',0,'ModeValue',-1,'DataType',0,'SLDataType','SS_DOUBLE','ByteLayout',0,'Factor',1,'Offset',0,'Min',0,'Max',255,'SgnComment',{{}},'SgnUnit',''),'MsgIdNumFormat',0,'MsgComment',{{''}}),'Version',1.2,'general',struct('isFromLib',1)),'GroupId',struct('Group',{{'RTICAN'}},'No',1,'Behavior',{{'NAMECHANGE'}},'BlockType',{{'SINK'}},'NameChangeFlag',0),'SFcnRTICANMessage',struct('MsgType','RX','MsgName',['RX Message'],'MsgIdFormat','STD','MsgId',100,'MsgLength',8,'NumSignals',1,'SampleTime',-1,'Signal',struct('SgnName',['RX signal'],'SgnStartBit',0,'SgnLength',8,'SgnType','standard','ModeValue',-1,'DataType',['unsigned int'],'ByteLayout',['little endian'],'SLDataType','SS_DOUBLE','Factor',1,'Offset',0),'StatusSelected','yes','TimeSelected','yes','DeltaTimeSelected','yes','BytePortSelected','no','MessageLengthSelected','no','EnablePortSelected','no','UserCoding',struct('Selected','no','InterfaceFile','UserDecodingFile','FcnName','UserDecodeFcn','InportSelected','no','InportWidth',1,'OutportSelected','no','OutportWidth',1),'TriggerPort',struct('Selected','no','TriggerType','rising'),'UseRXService','no','BoardType','DS4302','BoardNo',1,'ControllerNo',1,'SFcnPortType','Scalar'),'TLCFileName','rtican_rx_message')
      settings: AttributesFormatString=Group Id: RTICAN4\n
  Out1 : Outport
  wires:
  Bus Creator/1 -> Out1/1  "Track27"
  ESR_Track27/1 -> Bus Creator/1  "CAN_TX_TRACK_RANGE_RATE_27"
  ESR_Track27/2 -> Bus Creator/2  "CAN_TX_TRACK_MED_RANGE_MODE_27"
  ESR_Track27/3 -> Bus Creator/3  "CAN_TX_TRACK_RANGE_ACCEL_27"
  ESR_Track27/4 -> Bus Creator/4  "CAN_TX_TRACK_WIDTH_27"
  ESR_Track27/5 -> Bus Creator/5  "CAN_TX_TRACK_ROLLING_COUNT_27"
  ESR_Track27/6 -> Bus Creator/6  "CAN_TX_TRACK_BRIDGE_OBJECT_27"
  ESR_Track27/7 -> Bus Creator/7  "CAN_TX_TRACK_RANGE_27"
  ESR_Track27/8 -> Bus Creator/8  "CAN_TX_TRACK_ANGLE_27"
  ESR_Track27/9 -> Bus Creator/9  "CAN_TX_TRACK_STATUS_27"
  ESR_Track27/10 -> Bus Creator/10  "CAN_TX_TRACK_ONCOMING_27"
  ESR_Track27/11 -> Bus Creator/11  "CAN_TX_TRACK_GROUPING_CHANGED_27"
  ESR_Track27/12 -> Bus Creator/12  "CAN_TX_TRACK_LAT_RATE_27"

== system Control_test/InputProcessing/RadarCanProcessing/Track28 ==
  Bus Creator : BusCreator  Inputs=12
  ESR_Track28 : rtican/RTICAN Receive (RX)   Reserved1=[]  Reserved2=[]  Reserved3=[]  Reserved4=[]  SfcnMessage=[]  Msg_Struct=[]  BoardTypeNo=[]  BoardNo=[]  ChannelNo=[]  Parameters=[]  DialogFcn=[]  UnitName=[]  Revision=[]  UnitValues=[]  DSProperties=struct('RTI',struct('Version',uint32(5),'BlockType',struct('isSLSource',uint8(1),'isSLSink',uint8(1),'isHWSource',uint8(0),'isHWSink',uint8(0),'isSetup',uint8(0),'isInline',uint8(1),'isNonInline',uint8(0),'isInterrupt',uint8(0),'isChannelwise',uint8(0)),'IOBoardType','RTICAN','UnitType','MESSAGE','Identifier','RX','DialogType','MSVC','BlockSet','RTICAN','SlaveProcessor','CAN'))  RTIBlockInterface=struct('OutputPortsWidth',int32([1 1 1 1 1 1 1 1 1 1 1 1]),'OutputPortsActive',[1 1 1 1 1 1 1 1 1 1 1 1],'OutputPortsName',{{'CAN_TX_TRACK_RANGE_RATE_28','CAN_TX_TRACK_MED_RANGE_MODE_28','CAN_TX_TRACK_RANGE_ACCEL_28','CAN_TX_TRACK_WIDTH_28','CAN_TX_TRACK_ROLLING_COUNT_28','CAN_TX_TRACK_BRIDGE_OBJECT_28','CAN_TX_TRACK_RANGE_28','CAN_TX_TRACK_ANGLE_28','CAN_TX_TRACK_STATUS_28','CAN_TX_TRACK_ONCOMING_28','CAN_TX_TRACK_GROUPING_CHANGED_28','CAN_TX_TRACK_LAT_RATE_28'}},'OutputPortsDataType',{{'SS_DOUBLE','SS_DOUBLE','SS_DOUBLE','SS_DOUBLE','SS_DOUBLE','SS_DOUBLE','SS_DOUBLE','SS_DOUBLE','SS_DOUBLE','SS_DOUBLE','SS_DOUBLE','SS_DOUBLE'}},'OutputPortsLabel',{{'CAN_TX_TRACK_RANGE_RATE_28','CAN_TX_TRACK_MED_RANGE_MODE_28','CAN_TX_TRACK_RANGE_ACCEL_28','CAN_TX_TRACK_WIDTH_28','CAN_TX_TRACK_ROLLING_COUNT_28','CAN_TX_TRACK_BRIDGE_OBJECT_28','CAN_TX_TRACK_RANGE_28','CAN_TX_TRACK_ANGLE_28','CAN_TX_TRACK_STATUS_28','CAN_TX_TRACK_ONCOMING_28','CAN_TX_TRACK_GROUPING_CHANGED_28','CAN_TX_TRACK_LAT_RATE_28'}},'OutputPortsLabelMode','ON','InputPortsWidth',int32(0),'InputPortsActive',0,'DialogFcn','rtican_message_interface_gui','BlockDisplay',{{'','center'}},'IconTransparency','on','ParameterTunableNames',{{}},'InitLevel',3,'BlockName',struct('Token',{{'ESR_Track28'}}),'SampleTime',{{0.01}},'TriggerPort',{{'none'}},'EnablePort',{{'none'}})  RTIBlockParameters=struct('BoardTypeNo',{{1,'OFF',[]}},'BoardNo',{{2,'ON',[1 16]}},'ChannelNo',{{2,'ON',[1 2]}},'Parameters',{{struct('DataFileSupport',struct('DataFileSelectedMaster',1,'DataFileSelectedLocal',0,'DataFileName','c:\users\mpc_car\documents\github\mpc-car\controller\dbcfiles\esr_dv3_64tgt.dbc|','DataFileDate',{{{['02-Nov-2012 20:32:52']},{['21-Mar-2013 13:39:53']},{['28-Sep-2011 17:08:52']}}},'SelectedFile',['<no file selected>'],'InterfaceFcn','rtican_dbc_file_parser'),'Options',struct('StatusSelected',0,'TimeSelected',0,'DeltaTimeSelected',0,'BytePortSelected',0,'MessageLengthSelected',0,'TriggerPort',struct('Selected',0,'TriggerType',0),'UserCoding',struct('Selected',0,'InterfaceFile','UserDecodingFile','FcnName','UserDecodeFcn','InportSelected',0,'InportWidth',1,'OutportSelected',0,'OutportWidth',1),'EnablePortSelected',0,'SignalOnPortnameSelected',1,'UseRXService',0),'Message',struct('MsgOnBlocknameSelected',1,'MsgName','ESR_Track28','MsgIdFormat',0,'MsgId',1307,'MsgLength',8,'NumSignals',12,'SampleTime',0.01,'Signal',struct('SgnName',{'CAN_TX_TRACK_RANGE_RATE_28','CAN_TX_TRACK_MED_RANGE_MODE_28','CAN_TX_TRACK_RANGE_ACCEL_28','CAN_TX_TRACK_WIDTH_28','CAN_TX_TRACK_ROLLING_COUNT_28','CAN_TX_TRACK_BRIDGE_OBJECT_28','CAN_TX_TRACK_RANGE_28','CAN_TX_TRACK_ANGLE_28','CAN_TX_TRACK_STATUS_28','CAN_TX_TRACK_ONCOMING_28','CAN_TX_TRACK_GROUPING_CHANGED_28','CAN_TX_TRACK_LAT_RATE_28'},'SgnStartBit',{0,14,16,26,30,31,32,43,53,56,57,58},'SgnLength',{14,2,10,4,1,1,11,10,3,1,1,6},'SgnType',{0,0,0,0,0,0,0,0,0,0,0,0},'ModeValue',{-1,-1,-1,-1,-1,-1,-1,-1,-1,-1,-1,-1},'DataType',{1,0,1,0,0,0,0,1,0,0,0,1},'ByteLayout',{2,2,2,2,2,2,2,2,2,2,2,2},'Factor',{0.01,1,0.05,0.5,1,1,0.1,0.1,1,1,1,0.25},'Offset',{0,0,0,0,0,0,0,0,0,0,0,0},'SgnComment',{{''},{''},{''},{''},{''},{''},{''},{''},{''},{''},{''},{''}},'SgnUnit',{'m/s','','m/s/s','m','','','m','deg','','','',''},'Min',{-81.92,0,-25.6,0,0,0,0,-51.2,0,0,0,-8},'Max',{81.91,3,25.55,7.5,1,0,204.7,51.1,7,0,0,7.75},'SLDataType',{'SS_DOUBLE','SS_DOUBLE','SS_DOUBLE','SS_DOUBLE','SS_DOUBLE','SS_DOUBLE','SS_DOUBLE','SS_DOUBLE','SS_DOUBLE','SS_DOUBLE','SS_DOUBLE','SS_DOUBLE'}),'MsgIdNumFormat',0,'MsgComment',{{''}}),'Version',1.2,'general',struct('isFromLib',0)),'OFF',[]}},'GroupId',{{struct('Group',{{'RTICAN'}},'No',4,'Behavior',{{'NAMECHANGE'}},'BlockType',{{'SINK'}},'NameChangeFlag',0),'OFF',[]}},'SFcnRTICANMessage',{{struct('MsgType','RX','SFcnPortType','Scalar','MsgName','ESR_Track28','MsgIdFormat','STD','MsgId',1307,'MsgLength',8,'NumSignals',12,'SampleTime',0.01,'Signal',struct('SgnName',{'CAN_TX_TRACK_RANGE_RATE_28','CAN_TX_TRACK_MED_RANGE_MODE_28','CAN_TX_TRACK_RANGE_ACCEL_28','CAN_TX_TRACK_WIDTH_28','CAN_TX_TRACK_ROLLING_COUNT_28','CAN_TX_TRACK_BRIDGE_OBJECT_28','CAN_TX_TRACK_RANGE_28','CAN_TX_TRACK_ANGLE_28','CAN_TX_TRACK_STATUS_28','CAN_TX_TRACK_ONCOMING_28','CAN_TX_TRACK_GROUPING_CHANGED_28','CAN_TX_TRACK_LAT_RATE_28'},'SgnStartBit',{0,14,16,26,30,31,32,43,53,56,57,58},'SgnLength',{14,2,10,4,1,1,11,10,3,1,1,6},'SgnType',{'standard','standard','standard','standard','standard','standard','standard','standard','standard','standard','standard','standard'},'ModeValue',{-1,-1,-1,-1,-1,-1,-1,-1,-1,-1,-1,-1},'DataType',{['signed int'],['unsigned int'],['signed int'],['unsigned int'],['unsigned int'],['unsigned int'],['unsigned int'],['signed int'],['unsigned int'],['unsigned int'],['unsigned int'],['signed int']},'ByteLayout',{['motorola back.'],['motorola back.'],['motorola back.'],['motorola back.'],['motorola back.'],['motorola back.'],['motorola back.'],['motorola back.'],['motorola back.'],['motorola back.'],['motorola back.'],['motorola back.']},'Factor',{0.01,1,0.05,0.5,1,1,0.1,0.1,1,1,1,0.25},'Offset',{0,0,0,0,0,0,0,0,0,0,0,0},'SLDataType',{'SS_DOUBLE','SS_DOUBLE','SS_DOUBLE','SS_DOUBLE','SS_DOUBLE','SS_DOUBLE','SS_DOUBLE','SS_DOUBLE','SS_DOUBLE','SS_DOUBLE','SS_DOUBLE','SS_DOUBLE'}),'StatusSelected','no','TimeSelected','no','DeltaTimeSelected','no','BytePortSelected','no','MessageLengthSelected','no','TriggerPort',struct('Selected','no','TriggerType',0),'UserCoding',struct('Selected','no','InterfaceFile','UserDecodingFile','FcnName','UserDecodeFcn','InportSelected','no','InportWidth',1,'OutportSelected','no','OutportWidth',1),'EnablePortSelected','no','UseRXService','no','BoardType','DS1','BoardNo',2,'ControllerNo',2),'OFF',[]}},'TLCFileName',{{'rtican_rx_message','OFF',[]}})  RTISFcnParameters=struct('SFcnRTICANMessage','struct','TLCFileName','char')  RTIBlockParaDefault=struct('BoardTypeNo',4302,'BoardNo',1,'ChannelNo',1,'Parameters',struct('DataFileSupport',struct('DataFileSelectedMaster',0,'DataFileSelectedLocal',0,'DataFileName','','DataFileDate','','SelectedFile',['<no file selected>']),'Options',struct('StatusSelected',1,'TimeSelected',1,'DeltaTimeSelected',1,'BytePortSelected',0,'MessageLengthSelected',0,'TriggerPort',struct('Selected',0,'TriggerType','rising'),'UserCoding',struct('Selected',0,'InterfaceFile','UserDecodingFile','FcnName','UserDecodeFcn','InportSelected',0,'InportWidth',1,'OutportSelected',0,'OutportWidth',1),'EnablePortSelected',0,'SignalOnPortnameSelected',1,'UseRXService',0),'Message',struct('MsgOnBlocknameSelected',0,'MsgName',['RX Message'],'MsgIdFormat',0,'MsgId',100,'MsgLength',8,'NumSignals',1,'SampleTime',-1,'Signal',struct('SgnName',['RX signal'],'SgnStartBit',0,'SgnLength',8,'SgnType',0,'ModeValue',-1,'DataType',0,'SLDataType','SS_DOUBLE','ByteLayout',0,'Factor',1,'Offset',0,'Min',0,'Max',255,'SgnComment',{{}},'SgnUnit',''),'MsgIdNumFormat',0,'MsgComment',{{''}}),'Version',1.2,'general',struct('isFromLib',1)),'GroupId',struct('Group',{{'RTICAN'}},'No',1,'Behavior',{{'NAMECHANGE'}},'BlockType',{{'SINK'}},'NameChangeFlag',0),'SFcnRTICANMessage',struct('MsgType','RX','MsgName',['RX Message'],'MsgIdFormat','STD','MsgId',100,'MsgLength',8,'NumSignals',1,'SampleTime',-1,'Signal',struct('SgnName',['RX signal'],'SgnStartBit',0,'SgnLength',8,'SgnType','standard','ModeValue',-1,'DataType',['unsigned int'],'ByteLayout',['little endian'],'SLDataType','SS_DOUBLE','Factor',1,'Offset',0),'StatusSelected','yes','TimeSelected','yes','DeltaTimeSelected','yes','BytePortSelected','no','MessageLengthSelected','no','EnablePortSelected','no','UserCoding',struct('Selected','no','InterfaceFile','UserDecodingFile','FcnName','UserDecodeFcn','InportSelected','no','InportWidth',1,'OutportSelected','no','OutportWidth',1),'TriggerPort',struct('Selected','no','TriggerType','rising'),'UseRXService','no','BoardType','DS4302','BoardNo',1,'ControllerNo',1,'SFcnPortType','Scalar'),'TLCFileName','rtican_rx_message')
      settings: AttributesFormatString=Group Id: RTICAN4\n
  Out1 : Outport
  wires:
  Bus Creator/1 -> Out1/1  "Track28"
  ESR_Track28/1 -> Bus Creator/1  "CAN_TX_TRACK_RANGE_RATE_28"
  ESR_Track28/2 -> Bus Creator/2  "CAN_TX_TRACK_MED_RANGE_MODE_28"
  ESR_Track28/3 -> Bus Creator/3  "CAN_TX_TRACK_RANGE_ACCEL_28"
  ESR_Track28/4 -> Bus Creator/4  "CAN_TX_TRACK_WIDTH_28"
  ESR_Track28/5 -> Bus Creator/5  "CAN_TX_TRACK_ROLLING_COUNT_28"
  ESR_Track28/6 -> Bus Creator/6  "CAN_TX_TRACK_BRIDGE_OBJECT_28"
  ESR_Track28/7 -> Bus Creator/7  "CAN_TX_TRACK_RANGE_28"
  ESR_Track28/8 -> Bus Creator/8  "CAN_TX_TRACK_ANGLE_28"
  ESR_Track28/9 -> Bus Creator/9  "CAN_TX_TRACK_STATUS_28"
  ESR_Track28/10 -> Bus Creator/10  "CAN_TX_TRACK_ONCOMING_28"
  ESR_Track28/11 -> Bus Creator/11  "CAN_TX_TRACK_GROUPING_CHANGED_28"
  ESR_Track28/12 -> Bus Creator/12  "CAN_TX_TRACK_LAT_RATE_28"
